simulink model "RISE"  (R2018b)
settings: Solver=VariableStepAuto  StartTime=0.0  StopTime=sim_time  MaxStep=1e-3  RelTol=1e-3  AbsTol=1e-4
values from neighbouring files (symbols this model uses):
  W_hat_0 = 0.1*(rand(ctr_params.L,2)-0.5)    [RISE_params.m]    (also in RISE_virtualTest_params.m)
  x_0 = zeros(8,1)    [RISE_params.m]    (also in RISE_virtualTest_params.m = zeros(4,1))
  xi_0 = zeros(6,1)    [RISE_params.m]
undefined symbols (not defined in the file or in its folder): ctr_params
settings Model: Creator=RUZHOU  LastModifiedBy=RUZHOU

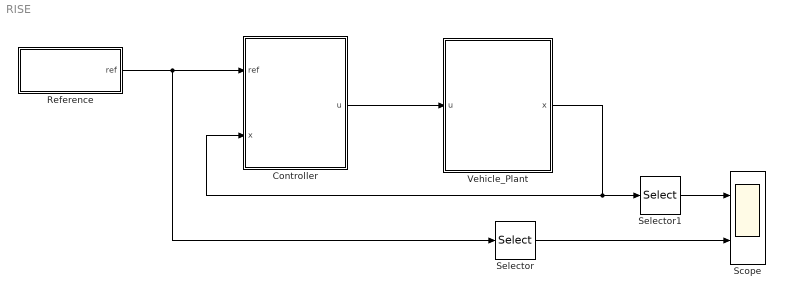
== system RISE ==
  Controller : Subsystem
  Reference : Subsystem
  Scope : Scope  NumInputPorts=2
  Selector : Selector  InputPortWidth=8  IndexOptions=Index vector (dialog)  Indices=[1 2]  OutputSizes=1
  Selector1 : Selector  InputPortWidth=8  IndexOptions=Index vector (dialog)  Indices=[1 2]  OutputSizes=1
  Vehicle_Plant : Subsystem
  wires:
  Controller/1(u) -> Vehicle_Plant/1(u)
  Selector1/1 -> Scope/1
  Vehicle_Plant/1(x) -> Selector1/1, Controller/2(x)
  Selector/1 -> Scope/2
  Reference/1(ref) -> Selector/1, Controller/1(ref)

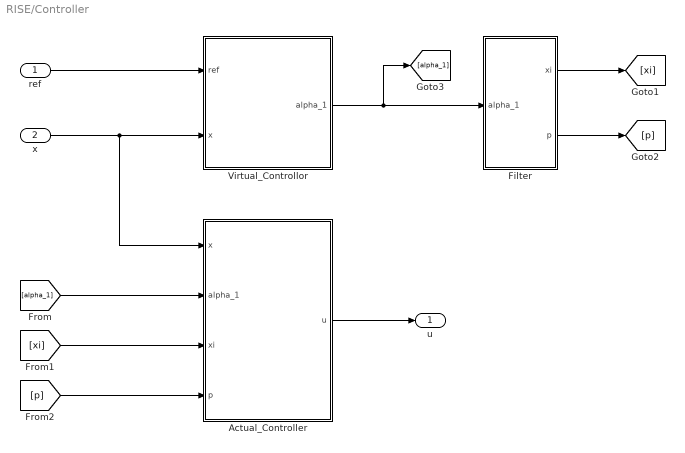
== system RISE/Controller ==
  ref : Inport
  x : Inport  Port=2
  Actual_Controller : Subsystem
  Filter : Subsystem
  Virtual_Controllor : Subsystem
  u : Outport
  wires:
  ref/1 -> Virtual_Controllor/1(ref)
  Virtual_Controllor/1(alpha_1) -> [alpha_1], Filter/1(alpha_1)
  x/1 -> Actual_Controller/1(x), Virtual_Controllor/2(x)
  Filter/1(xi) -> [xi]
  Filter/2(p) -> [p]
  [alpha_1] -> Actual_Controller/2(alpha_1)
  [xi] -> Actual_Controller/3(xi)
  [p] -> Actual_Controller/4(p)
  Actual_Controller/1(u) -> u/1

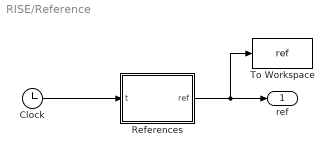
== system RISE/Reference ==
  Clock : Clock
  References : MATLAB Function  TreatAsAtomicUnit=on
  To Workspace : ToWorkspace  VariableName=ref  SaveFormat=Timeseries  SampleTime=-1
  ref : Outport
  wires:
  Clock/1 -> References/1(t)
  References/1(ref) -> To Workspace/1, ref/1

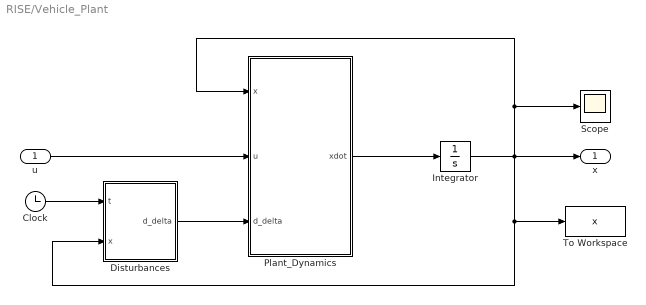
== system RISE/Vehicle_Plant ==
  u : Inport
  Clock : Clock
  Disturbances : MATLAB Function  TreatAsAtomicUnit=on
  Integrator : Integrator  InitialCondition=x_0
  Plant_Dynamics : MATLAB Function  TreatAsAtomicUnit=on
  Scope : Scope
  To Workspace : ToWorkspace  VariableName=x  SaveFormat=Timeseries  SampleTime=-1
  x : Outport
  wires:
  Disturbances/1(d_delta) -> Plant_Dynamics/3(d_delta)
  Clock/1 -> Disturbances/1(t)
  u/1 -> Plant_Dynamics/2(u)
  Plant_Dynamics/1(xdot) -> Integrator/1
  Integrator/1 -> To Workspace/1, Disturbances/2(x), Scope/1, Plant_Dynamics/1(x), x/1

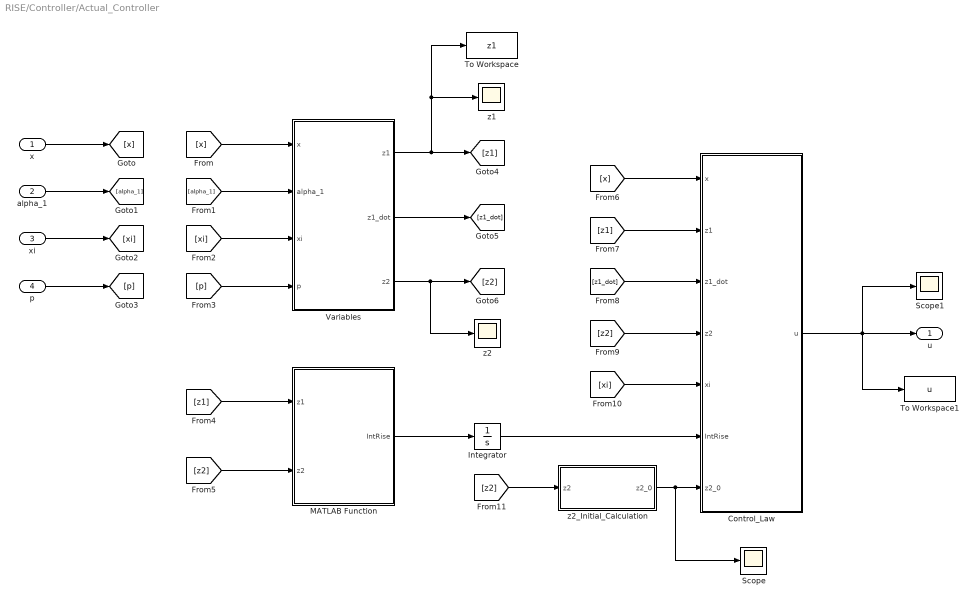
== system RISE/Controller/Actual_Controller ==
  x : Inport
  alpha_1 : Inport  Port=2
  xi : Inport  Port=3
  p : Inport  Port=4
  Control_Law : MATLAB Function  TreatAsAtomicUnit=on
  Integrator : Integrator  InitialCondition=zeros(2,1)
  MATLAB Function : MATLAB Function  TreatAsAtomicUnit=on
  Scope : Scope
  Scope1 : Scope
  To Workspace : ToWorkspace  VariableName=z1  SaveFormat=Timeseries  SampleTime=-1
  To Workspace1 : ToWorkspace  VariableName=u  SaveFormat=Timeseries  SampleTime=-1
  Variables : MATLAB Function  TreatAsAtomicUnit=on
  z1 : Scope
  z2 : Scope
  z2_Initial_Calculation : Subsystem
  u : Outport
  wires:
  x/1 -> [x]
  alpha_1/1 -> [alpha_1]
  xi/1 -> [xi]
  p/1 -> [p]
  [x] -> Variables/1(x)
  [alpha_1] -> Variables/2(alpha_1)
  [xi] -> Variables/3(xi)
  [p] -> Variables/4(p)
  Variables/1(z1) -> To Workspace/1, z1/1, [z1]
  Variables/2(z1_dot) -> [z1_dot]
  Variables/3(z2) -> z2/1, [z2]
  [z2] -> MATLAB Function/2(z2)
  [z1] -> MATLAB Function/1(z1)
  MATLAB Function/1(IntRise) -> Integrator/1
  Integrator/1 -> Control_Law/6(IntRise)
  [x] -> Control_Law/1(x)
  [z1] -> Control_Law/2(z1)
  [z1_dot] -> Control_Law/3(z1_dot)
  [z2] -> Control_Law/4(z2)
  Control_Law/1(u) -> To Workspace1/1, Scope1/1, u/1
  [xi] -> Control_Law/5(xi)
  [z2] -> z2_Initial_Calculation/1(z2)
  z2_Initial_Calculation/1(z2_0) -> Scope/1, Control_Law/7(z2_0)

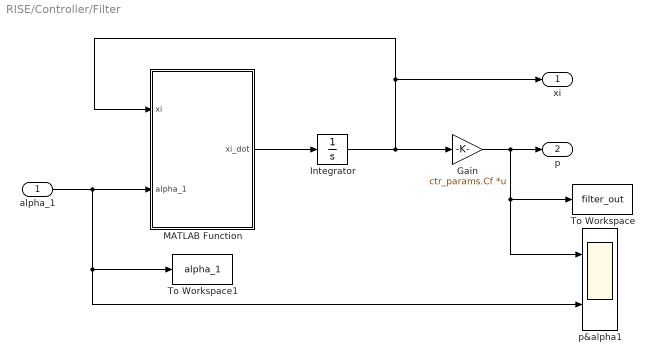
== system RISE/Controller/Filter ==
  alpha_1 : Inport
  Gain : Gain  Gain=ctr_params.Cf  Multiplication=Matrix(K*u)
  Integrator : Integrator  InitialCondition=xi_0
  MATLAB Function : MATLAB Function  TreatAsAtomicUnit=on
  To Workspace : ToWorkspace  VariableName=filter_out  SaveFormat=Timeseries  SampleTime=-1
  To Workspace1 : ToWorkspace  VariableName=alpha_1  SaveFormat=Timeseries  SampleTime=-1
  p&alpha1 : Scope  NumInputPorts=2
  xi : Outport
  p : Outport  Port=2
  wires:
  alpha_1/1 -> To Workspace1/1, p&alpha1/2, MATLAB Function/2(alpha_1)
  MATLAB Function/1(xi_dot) -> Integrator/1
  Integrator/1 -> Gain/1, MATLAB Function/1(xi), xi/1
  Gain/1 -> To Workspace/1, p&alpha1/1, p/1

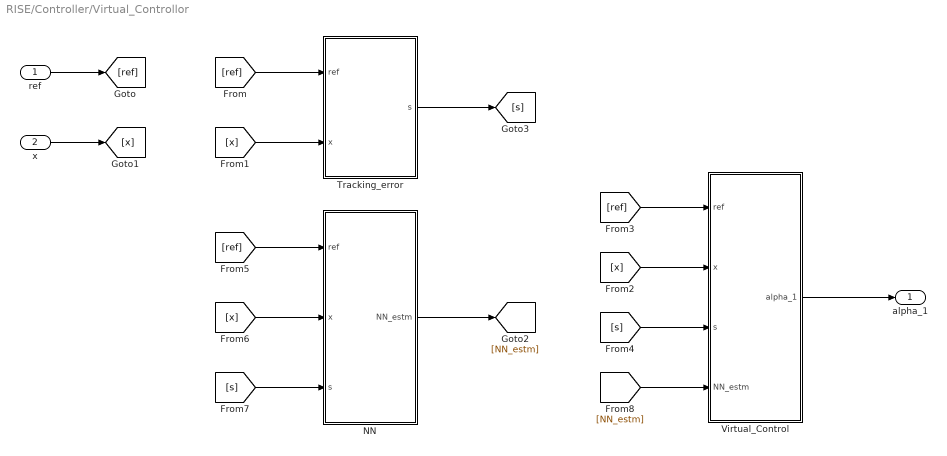
== system RISE/Controller/Virtual_Controllor ==
  ref : Inport
  x : Inport  Port=2
  NN : Subsystem
  Tracking_error : Subsystem
  Virtual_Control : Subsystem
  alpha_1 : Outport
  wires:
  [ref] -> Virtual_Control/1(ref)
  x/1 -> [x]
  ref/1 -> [ref]
  NN/1(NN_estm) -> [NN_estm]
  [NN_estm] -> Virtual_Control/4(NN_estm)
  [x] -> Virtual_Control/2(x)
  [x] -> NN/2(x)
  [s] -> NN/3(s)
  Tracking_error/1(s) -> [s]
  [s] -> Virtual_Control/3(s)
  [x] -> Tracking_error/2(x)
  [ref] -> Tracking_error/1(ref)
  [ref] -> NN/1(ref)
  Virtual_Control/1(alpha_1) -> alpha_1/1

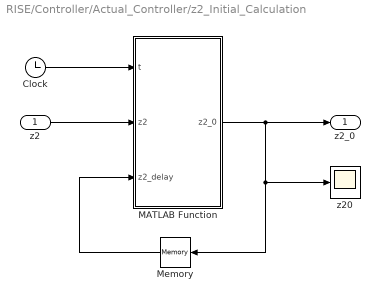
== system RISE/Controller/Actual_Controller/z2_Initial_Calculation ==
  z2 : Inport
  Clock : Clock
  MATLAB Function : MATLAB Function  TreatAsAtomicUnit=on
  Memory : Memory  InitialCondition=zeros(2,1)
  z20 : Scope
  z2_0 : Outport
  wires:
  z2/1 -> MATLAB Function/2(z2)
  Memory/1 -> MATLAB Function/3(z2_delay)
  MATLAB Function/1(z2_0) -> z2_0/1, z20/1, Memory/1
  Clock/1 -> MATLAB Function/1(t)

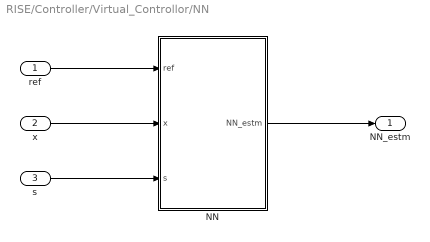
== system RISE/Controller/Virtual_Controllor/NN ==
  ref : Inport
  x : Inport  Port=2
  s : Inport  Port=3
  NN : Subsystem
  NN_estm : Outport
  wires:
  ref/1 -> NN/1(ref)
  x/1 -> NN/2(x)
  s/1 -> NN/3(s)
  NN/1(NN_estm) -> NN_estm/1

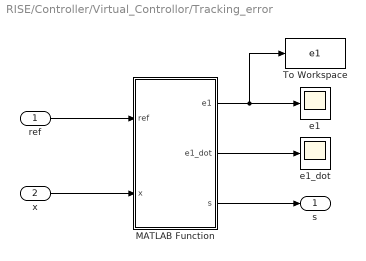
== system RISE/Controller/Virtual_Controllor/Tracking_error ==
  ref : Inport
  x : Inport  Port=2
  MATLAB Function : MATLAB Function  TreatAsAtomicUnit=on
  To Workspace : ToWorkspace  VariableName=e1  SaveFormat=Timeseries  SampleTime=-1
  e1 : Scope
  e1_dot : Scope
  s : Outport
  wires:
  MATLAB Function/2(e1_dot) -> e1_dot/1
  ref/1 -> MATLAB Function/1(ref)
  x/1 -> MATLAB Function/2(x)
  MATLAB Function/3(s) -> s/1
  MATLAB Function/1(e1) -> To Workspace/1, e1/1

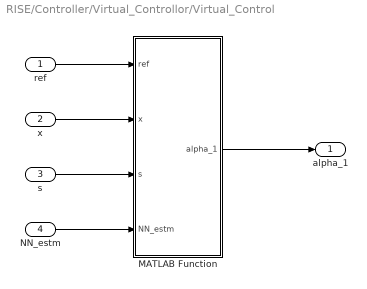
== system RISE/Controller/Virtual_Controllor/Virtual_Control ==
  ref : Inport
  x : Inport  Port=2
  s : Inport  Port=3
  NN_estm : Inport  Port=4
  MATLAB Function : MATLAB Function  TreatAsAtomicUnit=on
  alpha_1 : Outport
  wires:
  NN_estm/1 -> MATLAB Function/4(NN_estm)
  s/1 -> MATLAB Function/3(s)
  x/1 -> MATLAB Function/2(x)
  ref/1 -> MATLAB Function/1(ref)
  MATLAB Function/1(alpha_1) -> alpha_1/1

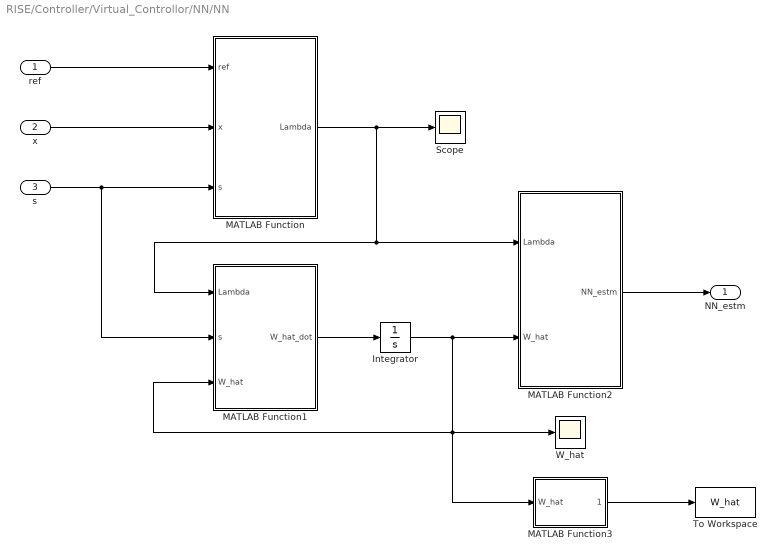
== system RISE/Controller/Virtual_Controllor/NN/NN ==
  ref : Inport
  x : Inport  Port=2
  s : Inport  Port=3
  Integrator : Integrator  InitialCondition=W_hat_0
  MATLAB Function : MATLAB Function  TreatAsAtomicUnit=on
  MATLAB Function1 : MATLAB Function  TreatAsAtomicUnit=on
  MATLAB Function2 : MATLAB Function  TreatAsAtomicUnit=on
  MATLAB Function3 : MATLAB Function  TreatAsAtomicUnit=on
  Scope : Scope
  To Workspace : ToWorkspace  VariableName=W_hat  SaveFormat=Timeseries  SampleTime=-1
  W_hat : Scope
  NN_estm : Outport
  wires:
  x/1 -> MATLAB Function/2(x)
  s/1 -> MATLAB Function/3(s), MATLAB Function1/2(s)
  ref/1 -> MATLAB Function/1(ref)
  MATLAB Function/1(Lambda) -> Scope/1, MATLAB Function1/1(Lambda), MATLAB Function2/1(Lambda)
  MATLAB Function1/1(W_hat_dot) -> Integrator/1
  Integrator/1 -> MATLAB Function3/1(W_hat), W_hat/1, MATLAB Function1/3(W_hat), MATLAB Function2/2(W_hat)
  MATLAB Function2/1(NN_estm) -> NN_estm/1
  MATLAB Function3/1(W_hat_norm) -> To Workspace/1

== matlab function RISE/Vehicle_Plant/Disturbances ==
  data: t input; d_delta output size=4; x input size=8
function d_delta = fcn(t,x)
% states
x1 = x(1:2); x3 = x(5:6); x4 = x(7:8);
d = 0.1*([15000;20000]*exp(-2*t)*sin(6*t)+5000*exp(-2*t)*x1);
delta = 0.1*([10;10]+30*x3 + [5;5]*(x4')*x4);
d_delta = [d;delta];
end

== matlab function RISE/Vehicle_Plant/Plant_Dynamics ==
  data: x input size=8; u input size=2; xdot output size=8; d_delta input size=4; sys_params parameter
function xdot = fcn(x,u,d_delta,sys_params)
% Parameters
G1 = sys_params.G1;
n1 = sys_params.n1;
s1 = sys_params.s1;
G2 = sys_params.G2;
n2 = sys_params.n2;
s2 = sys_params.s2;
eta = sys_params.eta;
l = sys_params.l;
L1 = sys_params.L1;
L2 = sys_params.L2;
L3 = sys_params.L3;
L4 = sys_params.L4;
m2 = sys_params.m2;
Jm1 = sys_params.Jm1;
Rm1 = sys_params.Rm1;
Ku1 = sys_params.Ku1;
K1 = sys_params.K1;
Ke1 = sys_params.Ke1;
Jm2 = sys_params.Jm2;
Rm2 = sys_params.Rm2;
Ku2 = sys_params.Ku2;
K2 = sys_params.K2;
Ke2 = sys_params.Ke2;
theta_1 = sys_params.theta_1;
theta_2 = sys_params.theta_2;
theta_3 = sys_params.theta_3;
C = sys_params.C;
g = sys_params.g;

%% States
x1 = x(1:2); x2 = x(3:4);
x3 = x(5:6); x4 = x(7:8);

%% Disturbance
d = d_delta(1:2);
delta = d_delta(3:4);

%% Nonlinear Functions
% Ma
Ma = zeros(2,2);
Ma(1,1) = 2547 + 5400*(sin(x1(2)))^2 - 2*sin(x1(2))*cos(x1(2)) + 224*(cos(x1(2)))^2;
Ma(1,2) = 2.8*sin(x1(2)) + 13.7*cos(x1(2));
Ma(2,1) = Ma(1,2);
Ma(2,2) = 5343;
% Mb
Mb = zeros(2,2);
Mb(1,2) = (10350*cos(x1(2))*sin(x1(2)) + 1.5*((cos(x1(2)))^2-(sin(x1(2)))^2))*x2(1)...
    - (13.7*sin(x1(2)) - 2.8*cos(x1(2)))*x2(2);
Mb(2,1) = -1/2*Mb(1,2);
Mb(2,2) = (1.5*cos(x1(2)) - 6.8*sin(x1(2)))*x2(1);
% W1
q0 = atan(L1/L2);
xp1 = sqrt(L3^2 + L1^2 + L2^2 - 2*L3*sqrt(L1^2+L2^2)*cos(x1(2)+q0));
h12 = L3*sqrt(L1^2+L2^2)*sin(x1(2)+q0)/xp1;
W1 = diag([G1/n1,2*pi*eta*G2/(n2*l)*h12]);
% W2
W2 = diag([G2,2*pi*eta*G2/l*h12]);
% W3
delta_q1 = x3(1)/n1 - x1(1);
delta_q2 = x3(2)/n2 - x1(2);
mu_1 = -2*s1*tanh(delta_q1/(2*s1));
mu_2 = -2*s2*tanh(delta_q2/(2*s2));
W3 = [mu_1;mu_2];
% W4
W4 = diag([K1*Ku1/(Jm1*Rm1),K2*Ku2/(Jm2*Rm2)]);
% W5
W5 = diag([Ke1*Ku1/(Jm1*Rm1),Ke2*Ku2/(Jm2*Rm2)]);
% W6
W6 = diag([1/n1,1/n2])*W1;
% W7
W7 = diag([1/n1,1/n2])*W2;
% W8
W8 = diag([1/n1,1/n2])*W3;
% Mg
Mg = [0;m2*g*L4*cos(x1(2))];

% phi
phi_1 = diag([tanh(C(1,1)*x2(1)),tanh(C(1,2)*x2(2))]);
phi_2 = diag([tanh(C(2,1)*x2(1))-tanh(C(3,1)*x2(1)),tanh(C(2,2)*x2(2))-tanh(C(3,2)*x2(2))]);
phi_3 = diag([x2(1),x2(2)]);
phi = [phi_1;phi_2;phi_3];
% theta
theta = [theta_1;theta_2;theta_3];

%% Dynamics
x1dot = x2;
x2dot = Ma\(W1*x3 - W2*x1 + W3 - Mb*x2 - (phi')*theta - Mg - d);
x3dot = x4;
x4dot = W4*u- W5*x4 -W6*x3 - W7*x1 + W8 - delta;

xdot = [x1dot;x2dot;x3dot;x4dot];
end

== matlab function RISE/Reference/References ==
  data: t input; ref output size=8
function ref = fcn(t)
% parameters
f1 = 0.2; a1 = 0.5; f2 = 0.08; a2 = 0.1;
x1d = [a1*sin(2*pi*f1*t);a2*sin(2*pi*f2*t)];
x1d_dot = [a1*2*pi*f1*cos(2*pi*f1*t);a2*2*pi*f2*cos(2*pi*f2*t)];
x1d_ddot = [-a1*(2*pi*f1)^2*sin(2*pi*f1*t);-a2*(2*pi*f2)^2*sin(2*pi*f2*t)];
x1d_3dot = [-a1*(2*pi*f1)^3*cos(2*pi*f1*t);-a2*(2*pi*f2)^3*cos(2*pi*f2*t)];
ref = [x1d;x1d_dot;x1d_ddot;x1d_3dot];
end

== matlab function RISE/Controller/Filter/MATLAB Function ==
  data: xi input size=6; xi_dot output size=6; alpha_1 input size=2; ctr_params parameter
function xi_dot = fcn(xi,alpha_1,ctr_params)
A = ctr_params.Af;
B = ctr_params.Bf;

xi_dot = A*xi + B*alpha_1;
end

== matlab function RISE/Controller/Actual_Controller/Variables ==
  data: x input size=8; z1 output size=2; alpha_1 input size=2; xi input size=6; p input size=2; z1_dot output size=2; z2 output size=2; ctr_params parameter
function [z1,z1_dot,z2] = fcn(x,alpha_1,xi,p,ctr_params)
% Parameters
A = ctr_params.Af;
B = ctr_params.Bf;
C = ctr_params.Cf;
sigma_2 = ctr_params.sigma_2;
% states
x3 = x(5:6); x4 = x(7:8);

%% variables
z1 = x3 - p;
z1_dot = x4 - C*(A*xi + B*alpha_1);
z2 = z1_dot + sigma_2*z1;

end

== matlab function RISE/Controller/Actual_Controller/MATLAB Function ==
  data: z1 input size=2; IntRise output size=2; z2 input size=2; ctr_params parameter
function IntRise = fcn(z1,z2,ctr_params)
% Parameters
Ks = ctr_params.Ks;
sigma_3 = ctr_params.sigma_3;
beta = ctr_params.beta;

%% Output
IntRise = Ks*(sigma_3*z2 + z1) + beta*sign(z2);
end

== matlab function RISE/Controller/Actual_Controller/Control_Law ==
  data: x input size=8; u output size=2; z1 input size=2; z1_dot input size=2; z2 input size=2; xi input size=6; IntRise input size=2; z2_0 input size=2; ctr_params parameter
function u = fcn(x,z1,z1_dot,z2,xi,IntRise,z2_0,ctr_params)
%% Parameters
% Nonimal plant
G1 = ctr_params.G1;
n1 = ctr_params.n1;
s1 = ctr_params.s1;
G2 = ctr_params.G2;
n2 = ctr_params.n2;
s2 = ctr_params.s2;
eta = ctr_params.eta;
l = ctr_params.l;
L1 = ctr_params.L1;
L2 = ctr_params.L2;
L3 = ctr_params.L3;
% L4 = ctr_params.L4;
% m2 = ctr_params.m2;
Jm1 = ctr_params.Jm1;
Rm1 = ctr_params.Rm1;
Ku1 = ctr_params.Ku1;
K1 = ctr_params.K1;
Ke1 = ctr_params.Ke1;
Jm2 = ctr_params.Jm2;
Rm2 = ctr_params.Rm2;
Ku2 = ctr_params.Ku2;
K2 = ctr_params.K2;
Ke2 = ctr_params.Ke2;
% theta_1 = ctr_params.theta_1;
% theta_2 = ctr_params.theta_2;
% theta_3 = ctr_params.theta_3;
% C = ctr_params.C;
% g = ctr_params.g;
% Actual control
Ks = ctr_params.Ks;
sigma_2 = ctr_params.sigma_2;
sigma_3 = ctr_params.sigma_3;

%% States
x1 = x(1:2);
x3 = x(5:6); x4 = x(7:8);
xi_3 = xi(5:6);

%% Nonlinear functions
% W1
q0 = atan(L1/L2);
xp1 = sqrt(L3^2 + L1^2 + L2^2 - 2*L3*sqrt(L1^2+L2^2)*cos(x1(2)+q0));
h12 = L3*sqrt(L1^2+L2^2)*sin(x1(2)+q0)/xp1;
W1 = diag([G1/n1,2*pi*eta*G2/(n2*l)*h12]);
% W2
W2 = diag([G2,2*pi*eta*G2/l*h12]);
% W3
delta_q1 = x3(1)/n1 - x1(1);
delta_q2 = x3(2)/n2 - x1(2);
mu_1 = -2*s1*tanh(delta_q1/(2*s1));
mu_2 = -2*s2*tanh(delta_q2/(2*s2));
W3 = [mu_1;mu_2];
% W4
W4 = diag([K1*Ku1/(Jm1*Rm1),K2*Ku2/(Jm2*Rm2)]);
% W5
W5 = diag([Ke1*Ku1/(Jm1*Rm1),Ke2*Ku2/(Jm2*Rm2)]);
% W6
W6 = diag([1/n1,1/n2])*W1;
% W7
W7 = diag([1/n1,1/n2])*W2;
% W8
W8 = diag([1/n1,1/n2])*W3;
% f2w
f2w = W4\(-W5*x4 - W6*x3 - W7*x1 + W8);
% Jw
Jw = W4\eye(2);
% nonlinear function F2
F2 = f2w + Jw*(sigma_2*z1_dot + sigma_3*z2 + z1 - xi_3);

%% Actual control laws
ur = -Ks*(z2 - z2_0) - IntRise;
u = ur + F2;
end

== matlab function RISE/Controller/Actual_Controller/z2_Initial_Calculation/MATLAB Function ==
  data: t input; z2_0 output; z2 input; z2_delay input
function z2_0 = fcn(t,z2,z2_delay)
if t == 0
    z2_0 = z2;
else
    z2_0 = z2_delay;
end
end

== matlab function RISE/Controller/Virtual_Controllor/NN/NN/MATLAB Function ==
  data: ref input size=8; Lambda output size=ctr_params.L; x input size=8; s input size=2; ctr_params parameter
function Lambda = fcn(ref,x,s,ctr_params)
% parameters
L = ctr_params.L;
c = ctr_params.c;
b = ctr_params.b;

% states
x1 = x(1:2); x2 = x(3:4); x3 = x(5:6);
x1d_dot = ref(3:4); x1d_ddot = ref(5:6);
e1_dot = x2 - x1d_dot;
Z = [x1;x2;x3;e1_dot;x1d_ddot;s];
Z_bar = [Z;1];

%% Gaussian Function
Lambda = zeros(L,1);
for i = 1:length(Lambda)
    Lambda(i,1) = exp(-((Z_bar-c(i))')*(Z_bar-c(i))/(2*b(i)^2));
end


end

== matlab function RISE/Controller/Virtual_Controllor/NN/NN/MATLAB Function1 ==
  data: Lambda input size=ctr_params.L; W_hat_dot output size=[ctr_params.L,2]; s input size=2; W_hat input size=[ctr_params.L,2]; ctr_params parameter
function W_hat_dot = fcn(Lambda,s,W_hat,ctr_params)
% parameters
gamma = ctr_params.gamma;
Gamma = ctr_params.Gamma;
Beta = ctr_params.Beta;
% Weight Update Law
W_hat_dot = gamma*Gamma*(Lambda*(s') - Beta*W_hat);
end

== matlab function RISE/Controller/Virtual_Controllor/NN/NN/MATLAB Function2 ==
  data: Lambda input size=ctr_params.L; NN_estm output size=2; W_hat input size=[ctr_params.L,2]
function NN_estm = fcn(Lambda,W_hat)

NN_estm = (W_hat')*Lambda;
end

== matlab function RISE/Controller/Virtual_Controllor/Tracking_error/MATLAB Function ==
  data: ref input size=8; e1 output size=2; x input size=8; e1_dot output size=2; s output size=2; ctr_params parameter
function [e1,e1_dot,s] = fcn(ref,x,ctr_params)
sigma_1 = ctr_params.sigma_1;
x1 = x(1:2); x2 = x(3:4);
x1d = ref(1:2); x1d_dot = ref(3:4);

e1 = x1 - x1d;
e1_dot = x2 - x1d_dot;
s = e1_dot + sigma_1*e1;
end

== matlab function RISE/Controller/Virtual_Controllor/Virtual_Control/MATLAB Function ==
  data: ref input size=8; alpha_1 output size=2; x input size=8; s input size=2; NN_estm input size=2; ctr_params parameter
function alpha_1 = fcn(ref,x,s,NN_estm,ctr_params)
%% parameters
% Nonimal plant
G1 = ctr_params.G1;
n1 = ctr_params.n1;
s1 = ctr_params.s1;
G2 = ctr_params.G2;
n2 = ctr_params.n2;
s2 = ctr_params.s2;
eta = ctr_params.eta;
l = ctr_params.l;
L1 = ctr_params.L1;
L2 = ctr_params.L2;
L3 = ctr_params.L3;
L4 = ctr_params.L4;
m2 = ctr_params.m2;
% Jm1 = ctr_params.Jm1;
% Rm1 = ctr_params.Rm1;
% Ku1 = ctr_params.Ku1;
% K1 = ctr_params.K1;
% Ke1 = ctr_params.Ke1;
% Jm2 = ctr_params.Jm2;
% Rm2 = ctr_params.Rm2;
% Ku2 = ctr_params.Ku2;
% K2 = ctr_params.K2;
% Ke2 = ctr_params.Ke2;
theta_1 = ctr_params.theta_1;
theta_2 = ctr_params.theta_2;
theta_3 = ctr_params.theta_3;
C = ctr_params.C;
g = ctr_params.g;
% Virtual control
sigma_1 = ctr_params.sigma_1;
rho = ctr_params.rho;
Kc1 = ctr_params.Kc1;
epsilon = ctr_params.epsilon;

%% states
x1 = x(1:2); x2 = x(3:4);
x3 = x(5:6);
x1d_dot = ref(3:4); x1d_ddot = ref(5:6);
e1_dot = x2 - x1d_dot;

%% Nominal functions
% Ma
Ma = zeros(2,2);
Ma(1,1) = 2547 + 5400*(sin(x1(2)))^2 - 2*sin(x1(2))*cos(x1(2)) + 224*(cos(x1(2)))^2;
Ma(1,2) = 2.8*sin(x1(2)) + 13.7*cos(x1(2));
Ma(2,1) = Ma(1,2);
Ma(2,2) = 5343;
% Mb
Mb = zeros(2,2);
Mb(1,2) = (10350*cos(x1(2))*sin(x1(2)) + 1.5*((cos(x1(2)))^2-(sin(x1(2)))^2))*x2(1)...
    - (13.7*sin(x1(2)) - 2.8*cos(x1(2)))*x2(2);
Mb(2,1) = -1/2*Mb(1,2);
Mb(2,2) = (1.5*cos(x1(2)) - 6.8*sin(x1(2)))*x2(1);
% W1
q0 = atan(L1/L2);
xp1 = sqrt(L3^2 + L1^2 + L2^2 - 2*L3*sqrt(L1^2+L2^2)*cos(x1(2)+q0));
h12 = L3*sqrt(L1^2+L2^2)*sin(x1(2)+q0)/xp1;
W1 = diag([G1/n1,2*pi*eta*G2/(n2*l)*h12]);
% W2
W2 = diag([G2,2*pi*eta*G2/l*h12]);
% W3
delta_q1 = x3(1)/n1 - x1(1);
delta_q2 = x3(2)/n2 - x1(2);
mu_1 = -2*s1*tanh(delta_q1/(2*s1));
mu_2 = -2*s2*tanh(delta_q2/(2*s2));
W3 = [mu_1;mu_2];
% Mg
Mg = [0;m2*g*L4*cos(x1(2))];
% phi
phi_1 = diag([tanh(C(1,1)*x2(1)),tanh(C(1,2)*x2(2))]);
phi_2 = diag([tanh(C(2,1)*x2(1))-tanh(C(3,1)*x2(1)),tanh(C(2,2)*x2(2))-tanh(C(3,2)*x2(2))]);
phi_3 = diag([x2(1),x2(2)]);
phi = [phi_1;phi_2;phi_3];
% theta
theta = [theta_1;theta_2;theta_3];

% Mw
Mw = W1\Ma;
% f1w
f1w = W1\(-W2*x1 + W3 - Mb*x2 - (phi')*theta - Mg);
% dMw_dt
dA11_dt = (5400*2*sin(x1(2))*cos(x1(2)) - 2*((cos(x1(2)))^2-(sin(x1(2)))^2) - 224*2*cos(x1(2))*sin(x1(2)))*x2(2);
dA12_dt = (2.8*cos(x1(2)) - 13.7*sin(x1(2)))*x2(2);
dA21_dt = dA12_dt;
dA22_dt = 0;
dxp1_dt = 1/2*(L3^2 + L1^2 + L2^2 - 2*L3*sqrt(L1^2+L2^2)*cos(x1(2)+q0))^(-1/2)*(2*L3*sqrt(L1^2+L2^2)*sin(x1(2)+q0))*x2(2);
dh12_dt = (L3*sqrt(L1^2+L2^2)*cos(x1(2)+q0)*x2(2)*xp1 - L3*sqrt(L1^2+L2^2)*sin(x1(2)+q0)*dxp1_dt)/(xp1^2);
dMw_dt = zeros(2,2);
dMw_dt(1,1) = n1/G1*dA11_dt;
dMw_dt(1,2) = n1/G1*dA12_dt;
dMw_dt(2,1) = l*n2/(2*pi*eta*G2)*(dA21_dt*h12-Ma(2,1)*dh12_dt)/(h12^2);
dMw_dt(2,2) = l*n2/(2*pi*eta*G2)*(dA22_dt*h12-Ma(2,2)*dh12_dt)/(h12^2);

F1 = f1w + Mw*(sigma_1*e1_dot-x1d_ddot) + 1/2*dMw_dt*s;

%% Contorl Law
alpha_1 = -F1 - Kc1*s - 1*NN_estm - 1*rho*tanh(s/epsilon);

end

== matlab function RISE/Controller/Virtual_Controllor/NN/NN/MATLAB Function3 ==
  data: W_hat input; W_hat_norm output
function W_hat_norm = fcn(W_hat)

W_hat_norm = norm(W_hat,2);
end
